simulink model "linear_acceleration"  (R2024b)
settings: Solver=VariableStepAuto  StartTime=0.0  StopTime=0.6  RelTol=1e-3
values from neighbouring files (symbols this model uses):
  tau = 0.1    [ex9.m]
settings Model: Creator=shohei  LastModifiedBy=shohei

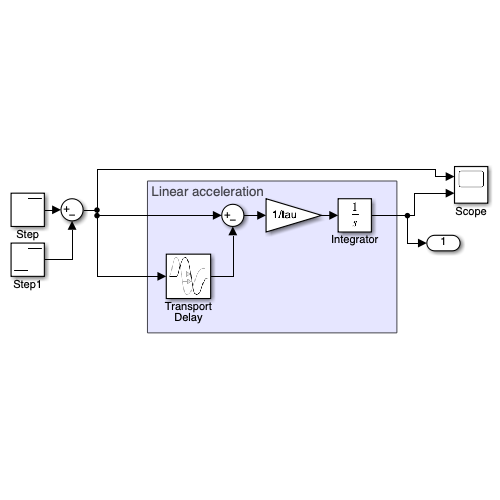
[thumbnail: Simulink's stored preview of the top-level diagram]
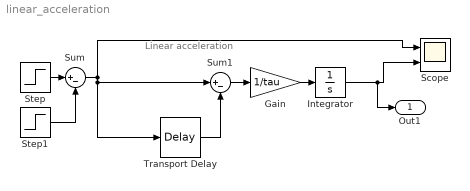
== system linear_acceleration ==
  note: Linear acceleration
  Gain : Gain  Gain=1/tau
  Integrator : Integrator
  Scope : Scope  NumInputPorts=2
  Step : Step  Time=0.1  SampleTime=0
  Step1 : Step  Time=0.4  SampleTime=0
  Sum : Sum  Inputs=|+-
  Sum1 : Sum  Inputs=|+-
  Transport Delay : TransportDelay  DelayTime=tau
  Out1 : Outport
  wires:
  Step1/1 -> Sum/2
  Step/1 -> Sum/1
  Sum1/1 -> Gain/1
  Sum/1 -> Scope/1, Transport Delay/1, Sum1/1
  Gain/1 -> Integrator/1
  Transport Delay/1 -> Sum1/2
  Integrator/1 -> Out1/1, Scope/2
